simulink model "TeamA_PAsqualo_R19b"  (R2019b)
settings: Solver=VariableStepAuto  StartTime=0.0  StopTime=stop_time  FixedStep=0.05  RelTol=1e-3
InitFcn:
  | main_init
values from neighbouring files (symbols this model uses):
  a1 = rho * D^4 * alpha1    (= 0.000388302366464)    [data_current.m]    (also in main_init.m)
  a2 = -rho * D^3 * alpha2 * (1 - omega)    (= 0.0037030698432)    [data_current.m]    (also in main_init.m)
  ag = [Ax Ay Az]'    [init_modello.m]
  alpha1 = 0.0113    [data_current.m]    (also in main_init.m)
  alpha2 = -0.0091    [data_current.m]    (also in main_init.m)
  areaOfInterestCorner = [42.317744;10.915136; 0]    [init_controllo.m]    (also in missionA.m = [42.317744)
  bg = [Bx By Bz]'    [init_modello.m]
  cd_pitch = 0.7    [init_modello.m]
  cd_roll = 0.04    [init_modello.m]
  cd_x = 0.4    [init_modello.m]
  cd_y = 1    [init_modello.m]
  cd_yaw = 0.7    [init_modello.m]
  cd_z = 1    [init_modello.m]
  cg = [Cx Cy Cz]'    [init_modello.m]
  D = 0.076    [data_current.m]    (also in main_init.m)
  dead_zone_limit = 31.5    [data_current.m]    (also in main_init.m)
  dg = [Dx Dy Dz]'    [init_modello.m]
  eg = [Ex Ey Ez]'    [init_modello.m]
  fg = [Fx Fy Fz]'    [init_modello.m]
  g = 9.81    [init_modello.m]
  galleggiamento = 66.5386    [init_controllo.m]
  gg = [Gx Gy Gz]'    [init_modello.m]
  H0 = 0    [init_modello.m]
  init_position = [pointP(1),pointP(2),0.15,0,0,deg2rad(angle)]'    [appunti.m]    (also in init_modello.m = [pointP(1),pointP(2),0.15,0,0,deg2rad(alpha)]')
  init_velocity = [0 0 0 0 0 0]'    [init_modello.m]
  initial_state_cov = blkdiag(diag(cov_gps(1,1:2)), cov_depth*eye(n_state_filter-2))    [init_navigazione.m]
  Ixx = 0.93304097392    [init_modello.m]
  Ixy = 0    [init_modello.m]
  Ixz = 0    [init_modello.m]
  Iyy = 25.58745481378    (= 25.5874548138)    [init_modello.m]
  Iyz = 0    [init_modello.m]
  Izz = 25.58745481378    (= 25.5874548138)    [init_modello.m]
  K_i_heave_div = 20    [init_controllo.m]
  K_i_heave_pos = 1    [init_controllo.m]
  K_i_heave_surf = 20    [init_controllo.m]
  K_i_heave_trans = 5    [init_controllo.m]
  K_i_heave_turn = 5    [init_controllo.m]
  K_i_pitch_div = 0    [init_controllo.m]
  K_i_pitch_pos = 0.1*0    (= 0)    [init_controllo.m]
  K_i_pitch_surf = 0    [init_controllo.m]
  K_i_pitch_trans = 0    [init_controllo.m]
  K_i_pitch_turn = 0    [init_controllo.m]
  K_i_roll_div = 0    [init_controllo.m]
  K_i_roll_pos = 0.1*0    (= 0)    [init_controllo.m]
  K_i_roll_surf = 1    [init_controllo.m]
  K_i_roll_trans = 0    [init_controllo.m]
  K_i_roll_turn = 0    [init_controllo.m]
  K_i_surge_div = 3    [init_controllo.m]
  K_i_surge_pos = 0.1679*30    (= 5.037)    [init_controllo.m]
  K_i_surge_surf = 3    [init_controllo.m]
  K_i_surge_trans = 0.1679*15    (= 2.5185)    [init_controllo.m]
  K_i_surge_turn = 0.1679*60    (= 10.074)    [init_controllo.m]
  K_i_sway_div = 6    [init_controllo.m]
  K_i_sway_pos = 5    [init_controllo.m]
  K_i_sway_surf = 3    [init_controllo.m]
  K_i_sway_trans = 2    [init_controllo.m]
  K_i_sway_turn = 50    [init_controllo.m]
  K_i_yaw_div = 0    [init_controllo.m]
  K_i_yaw_pos = 1    [init_controllo.m]
  K_i_yaw_surf = 0    [init_controllo.m]
  K_i_yaw_trans = 20    [init_controllo.m]
  K_p_heave_div = 200    [init_controllo.m]
  K_p_heave_pos = 320    [init_controllo.m]
  K_p_heave_surf = 200    [init_controllo.m]
  K_p_heave_trans = 170    [init_controllo.m]
  K_p_heave_turn = 170    [init_controllo.m]
  K_p_phi_div = 0.15    [init_controllo.m]
  K_p_phi_pos = 1*0.1    (= 0.1)    [init_controllo.m]
  K_p_phi_surf = 0.15    [init_controllo.m]
  K_p_phi_trans = 0.1    [init_controllo.m]
  K_p_phi_turn = 0.1    [init_controllo.m]
  K_p_pitch_div = 50    [init_controllo.m]
  K_p_pitch_pos = 25    [init_controllo.m]
  K_p_pitch_surf = 50    [init_controllo.m]
  K_p_pitch_trans = 25    [init_controllo.m]
  K_p_pitch_turn = 25    [init_controllo.m]
  K_p_psi_div = 0.3    [init_controllo.m]
  K_p_psi_pos = 0.25    [init_controllo.m]
  K_p_psi_surf = 0.3    [init_controllo.m]
  K_p_psi_trans = 0.2    [init_controllo.m]
  K_p_roll_div = 10    [init_controllo.m]
  K_p_roll_pos = 0.1*40    (= 4)    [init_controllo.m]
  K_p_roll_surf = 10    [init_controllo.m]
  K_p_roll_trans = 0.1*40    (= 4)    [init_controllo.m]
  K_p_roll_turn = 4    [init_controllo.m]
  K_p_surge_div = 80    [init_controllo.m]
  K_p_surge_pos = 13.7782*2.5    (= 34.4455)    [init_controllo.m]
  K_p_surge_surf = 80    [init_controllo.m]
  K_p_surge_trans = 20    [init_controllo.m]
  K_p_surge_turn = 150    [init_controllo.m]
  K_p_sway_div = 100    [init_controllo.m]
  K_p_sway_pos = 90    [init_controllo.m]
  K_p_sway_surf = 80    [init_controllo.m]
  K_p_sway_trans = 80    [init_controllo.m]
  K_p_sway_turn = 200    [init_controllo.m]
  K_p_th_div = 0.3    [init_controllo.m]
  K_p_th_pos = 0.1    [init_controllo.m]
  K_p_th_surf = 0.3    [init_controllo.m]
  K_p_th_trans = 0.1    [init_controllo.m]
  K_p_th_turn = 0.1    [init_controllo.m]
  K_p_x_div = 0.12    [init_controllo.m]
  K_p_x_pos = 0.12    [init_controllo.m]
  K_p_x_surf = 0.12    [init_controllo.m]
  K_p_y_div = 0.6    [init_controllo.m]
  K_p_y_pos = 0.34    [init_controllo.m]
  K_p_y_surf = 0.1    [init_controllo.m]
  K_p_y_trans = 0.3    [init_controllo.m]
  K_p_y_turn = 0.3    [init_controllo.m]
  K_p_yaw_div = 70    [init_controllo.m]
  K_p_yaw_pos = 20    [init_controllo.m]
  K_p_yaw_surf = 70    [init_controllo.m]
  K_p_yaw_trans = 160    [init_controllo.m]
  K_p_z_div = 0.35    [init_controllo.m]
  K_p_z_pos = 0.2    [init_controllo.m]
  K_p_z_surf = 0.35    [init_controllo.m]
  K_p_z_trans = 0.10    (= 0.1)    [init_controllo.m]
  K_p_z_turn = 0.1    [init_controllo.m]
  Kadd = 0    [init_modello.m]
  m = 100    [init_modello.m]    (also in retta.m = p2-p1)
  Madd = -((((1/5)*(b^2-a^2)^2))*(alpha_0-beta_0))/((((2*(b^2-a^2)^2))+(b^2-a^2)^2)*(alpha_0-beta_0)*m)    [init_modello.m]
  ... (+59 more)
undefined symbols (not defined in the file or in its folder): DiscIntNeverNeededParam, initial_state
libraries: simulink x2, vrlib x1
(part 1 of 6)
settings Model: PauseTimes=1  PacingRate=5  Creator=User  LastModifiedBy=tolom

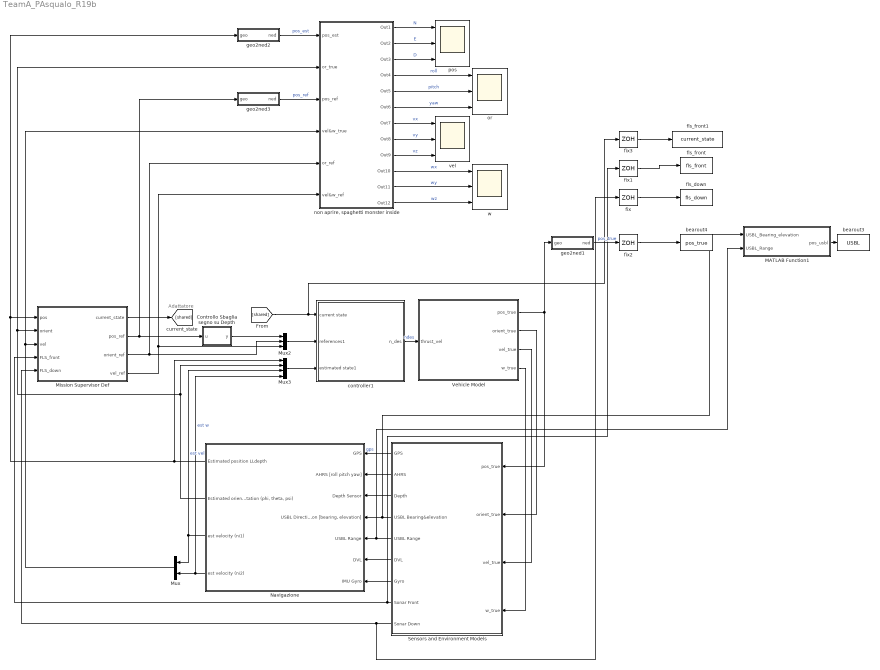
== system TeamA_PAsqualo_R19b ==
  note: Adattatore
  Controllo Sbaglia segno su Depth : MATLAB Function  TreatAsAtomicUnit=on
  MATLAB Function1 : MATLAB Function  TreatAsAtomicUnit=on
  Mission Supervisor Def : Subsystem
  Mux : Mux  Inputs=2
  Mux2 : Mux  Inputs=3
  Mux3 : Mux
  Navigazione : Subsystem
  "Sensors and Environment Models " : Subsystem
  Vehicle Model : Subsystem
  bearout3 : ToWorkspace  VariableName=USBL  SaveFormat=Structure With Time  SampleTime=-1
      settings: Save2DSignal=2-D array (concatenate along first dimension)
  bearout4 : ToWorkspace  VariableName=pos_true  SaveFormat=Structure With Time  SampleTime=-1
      settings: Save2DSignal=2-D array (concatenate along first dimension)
  controller1 : Subsystem
  fix{,1..3} (4 alike) : ZeroOrderHold  SampleTime=ts_filter
  fls_down : ToWorkspace  VariableName=fls_down  SaveFormat=Structure With Time  SampleTime=-1
      settings: Save2DSignal=2-D array (concatenate along first dimension)
  fls_front : ToWorkspace  VariableName=fls_front  SaveFormat=Structure With Time  SampleTime=-1
      settings: Save2DSignal=2-D array (concatenate along first dimension)
  fls_front1 : ToWorkspace  VariableName=current_state  SaveFormat=Structure With Time  SampleTime=-1
      settings: Save2DSignal=2-D array (concatenate along first dimension)
  geo2ned1 : MATLAB Function  TreatAsAtomicUnit=on
  geo2ned2 : MATLAB Function  TreatAsAtomicUnit=on
  geo2ned3 : MATLAB Function  TreatAsAtomicUnit=on
  "non aprire, spaghetti monster inside" : Subsystem
  or : Scope  NumInputPorts=3
  pos : Scope  NumInputPorts=3
  vel : Scope  NumInputPorts=3
  w : Scope  NumInputPorts=3
  wires:
  Mission Supervisor Def/4(vel_ref) -> "non aprire, spaghetti monster inside"/6(vel&w_ref), Mux2/3
  Mission Supervisor Def/3(orient_ref) -> "non aprire, spaghetti monster inside"/5(or_ref), Mux2/2
  Mission Supervisor Def/1(current_state) -> [shared]
  "Sensors and Environment Models "/8(Sonar Front) -> Mission Supervisor Def/4(FLS_front), fix1/1
  Vehicle Model/3(vel_true) -> "Sensors and Environment Models "/3(vel_true)
  Vehicle Model/4(w_true) -> "Sensors and Environment Models "/4(w_true)
  Mission Supervisor Def/2(pos_ref) -> geo2ned3/1(geo), Controllo Sbaglia segno su Depth/1(u)
  [shared] -> fix3/1, controller1/1(current state)
  Mux3/1 -> controller1/3(estimated state1)
  controller1/1(n_des) -> Vehicle Model/1(thrust_vel)  "ndes"
  "Sensors and Environment Models "/9(Sonar Down) -> Mission Supervisor Def/5(FLS_down), fix/1
  Vehicle Model/1(pos_true) -> "Sensors and Environment Models "/1(pos_true), geo2ned1/1(geo)
  Vehicle Model/2(orient_true) -> "Sensors and Environment Models "/2(orient_true)
  Navigazione/1(Estimated position LLdepth) -> Mux3/1, Mission Supervisor Def/1(pos), geo2ned2/1(geo)
  Navigazione/2("Estimated orientation (phi, theta, psi)") -> Mux3/2, Mission Supervisor Def/2(orient), "non aprire, spaghetti monster inside"/2(or_true)
  Navigazione/3(est velocity (ni1)) -> Mux/1, Mux3/3  "est vel"
  Navigazione/4(est velocity (ni2)) -> Mux3/4, Mux/2  "est w"
  Mux/1 -> Mission Supervisor Def/3(vel), "non aprire, spaghetti monster inside"/4(vel&w_true)
  geo2ned1/1(ned) -> fix2/1  "pos_true"
  MATLAB Function1/1(pos_usbl) -> bearout3/1
  "Sensors and Environment Models "/4(USBL Bearing&elevation) -> MATLAB Function1/1(USBL_Bearing_elevation), Navigazione/4("USBL Direction [bearing, elevation]")
  "Sensors and Environment Models "/5(USBL Range) -> MATLAB Function1/2(USBL_Range), Navigazione/5(USBL Range)
  "Sensors and Environment Models "/6(DVL) -> Navigazione/6(DVL)
  "Sensors and Environment Models "/7(Gyro) -> Navigazione/7(IMU Gyro)
  "Sensors and Environment Models "/3(Depth) -> Navigazione/3(Depth Sensor)
  "Sensors and Environment Models "/1(GPS) -> Navigazione/1(GPS)  "gps"
  "Sensors and Environment Models "/2(AHRS) -> Navigazione/2(AHRS [roll pitch yaw])
  "non aprire, spaghetti monster inside"/1(Out1) -> pos/1  "N"
  "non aprire, spaghetti monster inside"/2(Out2) -> pos/2  "E"
  "non aprire, spaghetti monster inside"/3(Out3) -> pos/3  "D"
  "non aprire, spaghetti monster inside"/4(Out4) -> or/1  "roll"
  "non aprire, spaghetti monster inside"/5(Out5) -> or/2  "pitch"
  "non aprire, spaghetti monster inside"/6(Out6) -> or/3  "yaw"
  "non aprire, spaghetti monster inside"/7(Out7) -> vel/1  "vx"
  "non aprire, spaghetti monster inside"/8(Out8) -> vel/2  "vy"
  "non aprire, spaghetti monster inside"/10(Out10) -> w/1  "wx"
  "non aprire, spaghetti monster inside"/11(Out11) -> w/2  "wy"
  "non aprire, spaghetti monster inside"/12(Out12) -> w/3  "wz"
  "non aprire, spaghetti monster inside"/9(Out9) -> vel/3  "vz"
  geo2ned2/1(ned) -> "non aprire, spaghetti monster inside"/1(pos_est)  "pos_est"
  geo2ned3/1(ned) -> "non aprire, spaghetti monster inside"/3(pos_ref)  "pos_ref"
  Mux2/1 -> controller1/2(references1)
  Controllo Sbaglia segno su Depth/1(y) -> Mux2/1
  fix/1 -> fls_down/1
  fix1/1 -> fls_front/1
  fix2/1 -> bearout4/1
  fix3/1 -> fls_front1/1

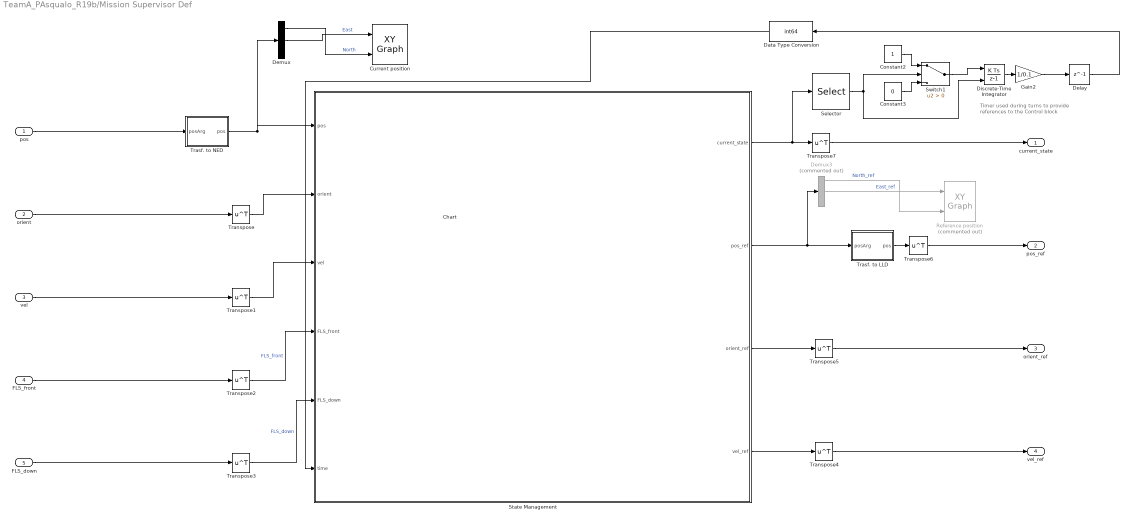
== system TeamA_PAsqualo_R19b/Mission Supervisor Def ==
  note: Timer used during turns to
      | provide references to the Control block
  pos : Inport
  orient : Inport  Port=2  PortDimensions=[3 1]
  vel : Inport  Port=3  PortDimensions=[6 1]
  FLS_front : Inport  Port=4  PortDimensions=1
  FLS_down : Inport  Port=5  PortDimensions=1
  Chart : Stateflow chart  TreatAsAtomicUnit=on
  Constant2 : Constant
  Constant3 : Constant  Value=0
  Current position : simulink/Sinks/XY Graph  xmin=0  xmax=150  ymin=0  ymax=150  st=-1
  Data Type Conversion : DataTypeConversion  OutDataTypeStr=int64
  Delay : Delay  DelayLength=1  SampleTime=0.1
  Demux : Demux  Outputs=3
  Demux3 : Demux  Commented=on  Outputs=3
  Discrete-Time Integrator : DiscreteIntegrator  ExternalReset=falling  SampleTime=0.1  ICPrevOutput=DiscIntNeverNeededParam  ICPrevScaledInput=DiscIntNeverNeededParam
  Gain2 : Gain  Gain=1/0.1
  Reference position : simulink/Sinks/XY Graph  Commented=on  xmin=0  xmax=150  ymin=0  ymax=150  st=-1
  Selector : Selector  InputPortWidth=8  IndexOptions=Index vector (dialog)  Indices=4  OutputSizes=1
  State Management : Stateflow chart  TreatAsAtomicUnit=on
  Switch1 : Switch  Criteria=u2 > Threshold
  Transpose{,1..7} (8 alike) : Math  Operator=transpose  SaturateOnIntegerOverflow=on
  Trasf. to LLD : MATLAB Function  TreatAsAtomicUnit=on
  Trasf. to NED : MATLAB Function  TreatAsAtomicUnit=on
  current_state : Outport
  pos_ref : Outport  Port=2
  orient_ref : Outport  Port=3
  vel_ref : Outport  Port=4  PortDimensions=[6 1]
  wires:
  Transpose3/1 -> State Management/5(FLS_down)  "FLS_down"
  FLS_front/1 -> Transpose2/1
  Transpose5/1 -> orient_ref/1
  orient/1 -> Transpose/1
  vel/1 -> Transpose1/1
  Transpose4/1 -> vel_ref/1
  FLS_down/1 -> Transpose3/1
  Demux/1 -> Current position/2  "North"
  Demux/2 -> Current position/1  "East"
  Transpose/1 -> State Management/2(orient)
  Transpose1/1 -> State Management/3(vel)
  Transpose2/1 -> State Management/4(FLS_front)  "FLS_front"
  Demux3/1 -> Reference position/2  "North_ref"
  Demux3/2 -> Reference position/1  "East_ref"
  State Management/3(orient_ref) -> Transpose5/1
  State Management/4(vel_ref) -> Transpose4/1
  pos/1 -> Trasf. to NED/1(posArg)
  State Management/2(pos_ref) -> Trasf. to LLD/1(posArg), Demux3/1
  Trasf. to LLD/1(pos) -> Transpose6/1
  Trasf. to NED/1(pos) -> Demux/1, State Management/1(pos)
  Transpose6/1 -> pos_ref/1
  Transpose7/1 -> current_state/1
  Discrete-Time Integrator/1 -> Gain2/1
  Selector/1 -> Discrete-Time Integrator/2, Switch1/2
  Switch1/1 -> Discrete-Time Integrator/1
  Constant3/1 -> Switch1/3
  Constant2/1 -> Switch1/1
  Data Type Conversion/1 -> State Management/6(time)
  Gain2/1 -> Delay/1
  Delay/1 -> Data Type Conversion/1
  State Management/1(current_state) -> Selector/1, Transpose7/1

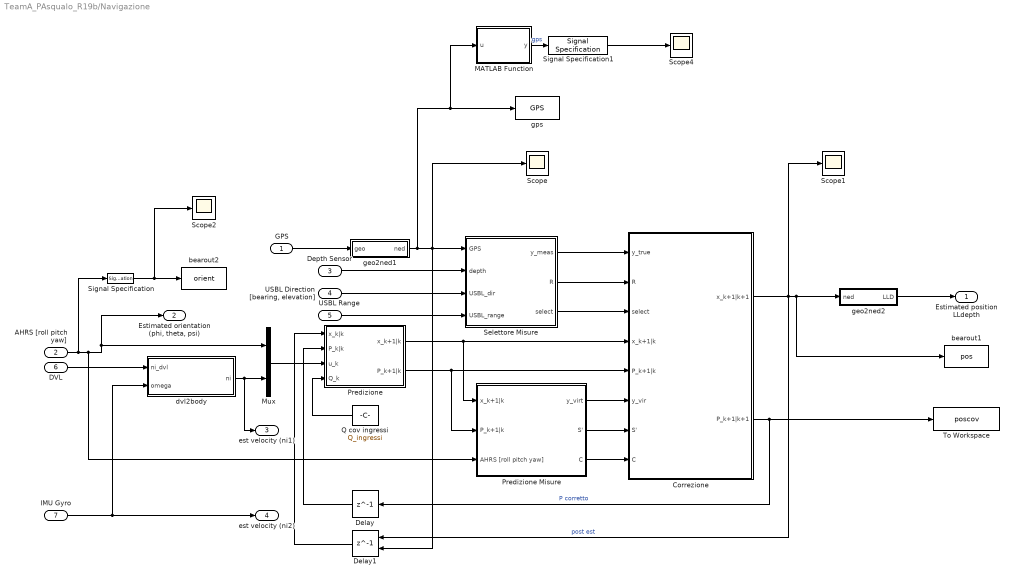
== system TeamA_PAsqualo_R19b/Navigazione ==
  GPS : Inport  PortDimensions=[3 1]
  AHRS [roll pitch yaw] : Inport  Port=2  PortDimensions=[3 1]
  Depth Sensor : Inport  Port=3  PortDimensions=[1 1]
  "USBL Direction [bearing, elevation]" : Inport  Port=4  PortDimensions=[2 1]
  USBL Range : Inport  Port=5  PortDimensions=[1 1]
  DVL : Inport  Port=6  PortDimensions=[3 1]
  IMU Gyro : Inport  Port=7  PortDimensions=[3 1]
  Correzione : Subsystem
  Delay : Delay  DelayLength=1  InitialCondition=initial_state_cov  SampleTime=ts_filter
  Delay1 : Delay  DelayLength=1  InitialConditionSource=Input port  InitialCondition=initial_state  SampleTime=ts_filter
      settings: InputPortMap=u0,p4
  MATLAB Function : MATLAB Function  TreatAsAtomicUnit=on
  Mux : Mux  Inputs=2
  Predizione : Subsystem
  Predizione Misure : Subsystem
  Q cov ingressi : Constant  Value=Q_ingressi
  Scope{,1..2,4} (4 alike) : Scope
  Selettore Misure : Subsystem
  Signal Specification : SignalSpecification  Dimensions=[3,1]
  Signal Specification1 : SignalSpecification  Dimensions=1
  To Workspace : ToWorkspace  VariableName=poscov  SaveFormat=Structure With Time  SampleTime=-1
  bearout1 : ToWorkspace  VariableName=pos  SaveFormat=Structure With Time  SampleTime=-1
      settings: Save2DSignal=2-D array (concatenate along first dimension)
  bearout2 : ToWorkspace  VariableName=orient  SaveFormat=Structure With Time  SampleTime=-1
      settings: Save2DSignal=2-D array (concatenate along first dimension)
  dvl2body : MATLAB Function  TreatAsAtomicUnit=on
  geo2ned1 : MATLAB Function  TreatAsAtomicUnit=on
  geo2ned2 : MATLAB Function  TreatAsAtomicUnit=on
  gps : ToWorkspace  VariableName=GPS  SaveFormat=Structure With Time  SampleTime=-1
      settings: Save2DSignal=2-D array (concatenate along first dimension)
  Estimated position LLdepth : Outport
  "Estimated orientation (phi, theta, psi)" : Outport  Port=2
  est velocity (ni1) : Outport  Port=3
  est velocity (ni2) : Outport  Port=4
  wires:
  Delay1/1 -> Predizione/1(x_k|k)
  Selettore Misure/2(R) -> Correzione/2(R)
  Selettore Misure/1(y_meas) -> Correzione/1(y_true)
  USBL Range/1 -> Selettore Misure/4(USBL_range)
  DVL/1 -> dvl2body/1(ni_dvl)
  Correzione/2(P_k+1|k+1) -> Delay/1, To Workspace/1  "P corretto"
  Predizione Misure/3(C) -> Correzione/8(C)
  Mux/1 -> Predizione/3(u_k)
  GPS/1 -> geo2ned1/1(geo)
  dvl2body/1(ni) -> est velocity (ni1)/1, Mux/2
  Delay/1 -> Predizione/2(P_k|k)
  Selettore Misure/3(select) -> Correzione/3(select)
  Depth Sensor/1 -> Selettore Misure/2(depth)
  Predizione Misure/2(S') -> Correzione/7(S')
  "USBL Direction [bearing, elevation]"/1 -> Selettore Misure/3(USBL_dir)
  Q cov ingressi/1 -> Predizione/4(Q_k)
  Predizione/1(x_k+1|k) -> Predizione Misure/1(x_k+1|k), Correzione/4(x_k+1|k)
  Predizione Misure/1(y_virt) -> Correzione/6(y_vir)
  AHRS [roll pitch yaw]/1 -> Predizione Misure/3(AHRS [roll pitch yaw]), Mux/1, "Estimated orientation (phi, theta, psi)"/1, Signal Specification/1
  Predizione/2(P_k+1|k) -> Predizione Misure/2(P_k+1|k), Correzione/5(P_k+1|k)
  IMU Gyro/1 -> est velocity (ni2)/1, dvl2body/2(omega)
  geo2ned2/1(LLD) -> Estimated position LLdepth/1
  Correzione/1(x_k+1|k+1) -> Scope1/1, bearout1/1, geo2ned2/1(ned), Delay1/1  "post est"
  Signal Specification/1 -> Scope2/1, bearout2/1
  geo2ned1/1(ned) -> MATLAB Function/1(u), gps/1, Scope/1, Delay1/2, Selettore Misure/1(GPS)
  MATLAB Function/1(y) -> Signal Specification1/1  "gps"
  Signal Specification1/1 -> Scope4/1

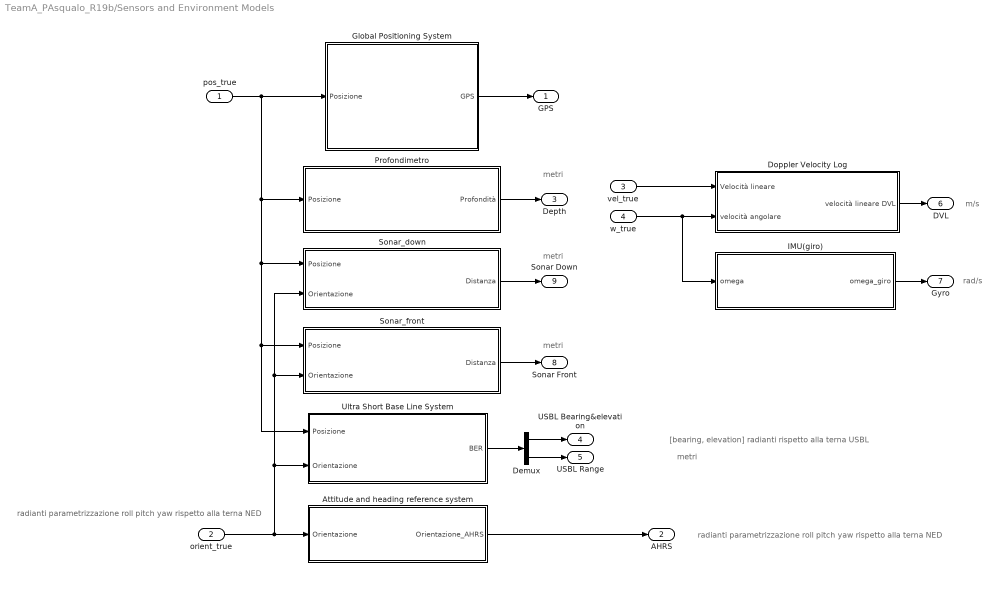
== system TeamA_PAsqualo_R19b/Sensors and Environment Models  ==
  note: radianti parametrizzazione roll pitch yaw rispetto alla terna NED
  note: m/s
  note: metri
  note: [bearing, elevation] radianti rispetto alla terna USBL
  note: rad/s
  note: metri
  note: metri
  note: metri
  note: radianti parametrizzazione roll pitch yaw rispetto alla terna NED
  pos_true : Inport
  orient_true : Inport  Port=2
  vel_true : Inport  Port=3
  w_true : Inport  Port=4
  Attitude and heading reference system : Subsystem
  Demux : Demux  Outputs=2
  Doppler Velocity Log : Subsystem
  Global Positioning System : Subsystem
  IMU(giro) : Subsystem
  Profondimetro : Subsystem
  Sonar_down : Subsystem
  Sonar_front : Subsystem
  Ultra Short Base Line System : Subsystem
  GPS : Outport
  AHRS : Outport  Port=2
  Depth : Outport  Port=3
  USBL Bearing&elevation : Outport  Port=4
  USBL Range : Outport  Port=5
  DVL : Outport  Port=6
  Gyro : Outport  Port=7
  Sonar Front : Outport  Port=8
  Sonar Down : Outport  Port=9
  wires:
  IMU(giro)/1(omega_giro) -> Gyro/1
  vel_true/1 -> Doppler Velocity Log/1(Velocità lineare)
  pos_true/1 -> Ultra Short Base Line System/1(Posizione), Sonar_front/1(Posizione), Sonar_down/1(Posizione), Profondimetro/1(Posizione), Global Positioning System/1(Posizione)
  orient_true/1 -> Attitude and heading reference system/1(Orientazione), Ultra Short Base Line System/2(Orientazione), Sonar_down/2(Orientazione), Sonar_front/2(Orientazione)
  w_true/1 -> IMU(giro)/1(omega), Doppler Velocity Log/2(velocità angolare)
  Sonar_down/1(Distanza) -> Sonar Down/1
  Profondimetro/1(Profondità) -> Depth/1
  Demux/2 -> USBL Range/1
  Doppler Velocity Log/1(velocità lineare DVL) -> DVL/1
  Sonar_front/1(Distanza) -> Sonar Front/1
  Global Positioning System/1(GPS) -> GPS/1
  Demux/1 -> USBL Bearing&elevation/1
  Attitude and heading reference system/1(Orientazione_AHRS) -> AHRS/1
  Ultra Short Base Line System/1(BER) -> Demux/1

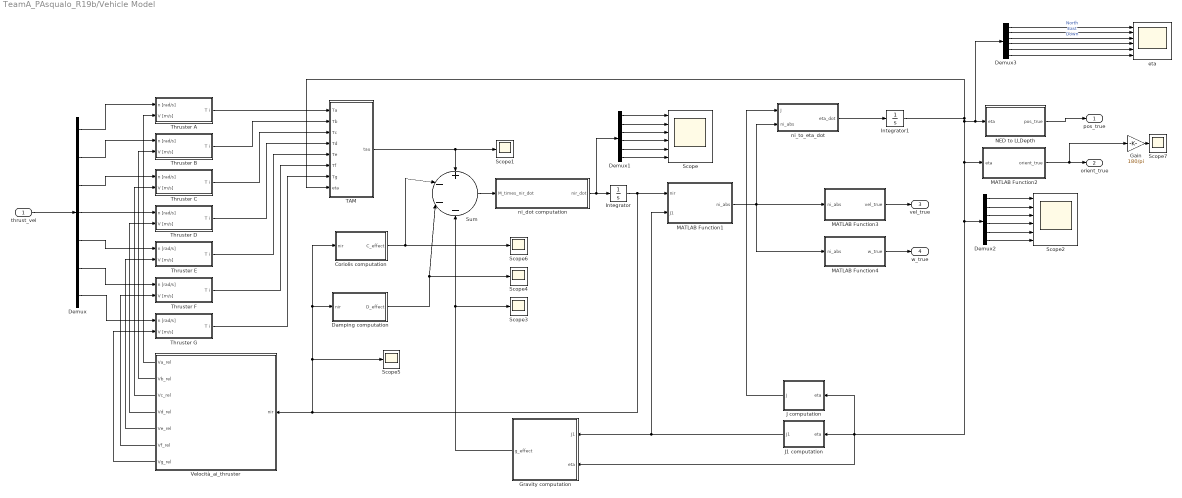
== system TeamA_PAsqualo_R19b/Vehicle Model ==
  thrust_vel : Inport
  Coriolis computation : MATLAB Function  TreatAsAtomicUnit=on
  Damping computation : MATLAB Function  TreatAsAtomicUnit=on
  Demux : Demux  Outputs=7
  Demux1 : Demux  Outputs=6
  Demux2 : Demux  Outputs=6
  Demux3 : Demux  Outputs=6
  Gain : Gain  Gain=180/pi
  Gravity computation : MATLAB Function  TreatAsAtomicUnit=on
  Integrator : Integrator  InitialCondition=init_velocity  ContinuousStateAttributes='velocity'
  Integrator1 : Integrator  InitialCondition=init_position  ContinuousStateAttributes='position'
  J computation : MATLAB Function  TreatAsAtomicUnit=on
  J1 computation : MATLAB Function  TreatAsAtomicUnit=on
  MATLAB Function1 : MATLAB Function  TreatAsAtomicUnit=on
  MATLAB Function2 : MATLAB Function  TreatAsAtomicUnit=on
  MATLAB Function3 : MATLAB Function  TreatAsAtomicUnit=on
  MATLAB Function4 : MATLAB Function  TreatAsAtomicUnit=on
  NED to LLDepth : MATLAB Function  TreatAsAtomicUnit=on
  Scope : Scope  NumInputPorts=6
  Scope{1,3..7} (6 alike) : Scope
  Scope2 : Scope  NumInputPorts=6
  Sum : Sum  Inputs=+---
  TAM : MATLAB Function
  Thruster A : Subsystem
  Thruster B : Subsystem
  Thruster C : Subsystem
  Thruster D : Subsystem
  Thruster E : Subsystem
  Thruster F : Subsystem
  Thruster G : Subsystem
  Velocità_ai_thruster : MATLAB Function  TreatAsAtomicUnit=on
  eta : Scope  NumInputPorts=6
  ni_dot computation : MATLAB Function  TreatAsAtomicUnit=on
  ni_to_eta_dot : MATLAB Function  TreatAsAtomicUnit=on
  pos_true : Outport
  orient_true : Outport  Port=2
  vel_true : Outport  Port=3
  w_true : Outport  Port=4
  wires:
  Demux/3 -> Thruster C/1(n [rad/s])
  Thruster A/1(T i) -> TAM/1(Ta)
  Thruster G/1(T i) -> TAM/7(Tg)
  Sum/1 -> ni_dot computation/1(M_times_nir_dot)
  Velocità_ai_thruster/7(Vg_rel) -> Thruster G/2(V [m/s])
  Velocità_ai_thruster/3(Vc_rel) -> Thruster C/2(V [m/s])
  Thruster C/1(T i) -> TAM/3(Tc)
  MATLAB Function3/1(vel_true) -> vel_true/1
  Gravity computation/1(g_effect) -> Sum/4, Scope3/1
  Demux/6 -> Thruster F/1(n [rad/s])
  MATLAB Function4/1(w_true) -> w_true/1
  J1 computation/1(J1) -> Gravity computation/1(J1), MATLAB Function1/2(J1)
  Thruster F/1(T i) -> TAM/6(Tf)
  Integrator/1 -> Scope5/1, Coriolis computation/1(nir), Damping computation/1(nir), Velocità_ai_thruster/1(nir), MATLAB Function1/1(nir)
  Velocità_ai_thruster/4(Vd_rel) -> Thruster D/2(V [m/s])
  Velocità_ai_thruster/6(Vf_rel) -> Thruster F/2(V [m/s])
  ni_dot computation/1(nir_dot) -> Demux1/1, Integrator/1
  Velocità_ai_thruster/2(Vb_rel) -> Thruster B/2(V [m/s])
  MATLAB Function1/1(ni_abs) -> ni_to_eta_dot/2(ni_abs), MATLAB Function3/1(ni_abs), MATLAB Function4/1(ni_abs)
  Velocità_ai_thruster/1(Va_rel) -> Thruster A/2(V [m/s])
  Demux/4 -> Thruster D/1(n [rad/s])
  Thruster E/1(T i) -> TAM/5(Te)
  Thruster B/1(T i) -> TAM/2(Tb)
  Demux/2 -> Thruster B/1(n [rad/s])
  TAM/1(tau) -> Sum/1, Scope1/1
  ni_to_eta_dot/1(eta_dot) -> Integrator1/1
  MATLAB Function2/1(orient_true) -> Gain/1, orient_true/1
  Demux/1 -> Thruster A/1(n [rad/s])
  Velocità_ai_thruster/5(Ve_rel) -> Thruster E/2(V [m/s])
  Demux/5 -> Thruster E/1(n [rad/s])
  NED to LLDepth/1(pos_true) -> pos_true/1
  Thruster D/1(T i) -> TAM/4(Td)
  J computation/1(J) -> ni_to_eta_dot/1(J)
  thrust_vel/1 -> Demux/1
  Demux/7 -> Thruster G/1(n [rad/s])
  Damping computation/1(D_effect) -> Sum/3, Scope4/1
  Coriolis computation/1(C_effect) -> Sum/2, Scope6/1
  Demux1/1 -> Scope/1
  Demux1/2 -> Scope/2
  Demux1/3 -> Scope/3
  Demux1/5 -> Scope/5
  Demux1/6 -> Scope/6
  Demux1/4 -> Scope/4
  Demux2/6 -> Scope2/6
  Demux2/5 -> Scope2/5
  Demux2/3 -> Scope2/3
  Demux2/2 -> Scope2/2
  Demux2/4 -> Scope2/4
  Demux2/1 -> Scope2/1
  Demux3/3 -> eta/3  "Down"
  Demux3/1 -> eta/1  "North"
  Demux3/2 -> eta/2  "East"
  Integrator1/1 -> TAM/8(eta), Demux3/1, NED to LLDepth/1(eta), J computation/1(eta), Gravity computation/2(eta), J1 computation/1(eta), Demux2/1, MATLAB Function2/1(eta)
  Demux3/4 -> eta/4
  Demux3/5 -> eta/5
  Demux3/6 -> eta/6
  Gain/1 -> Scope7/1

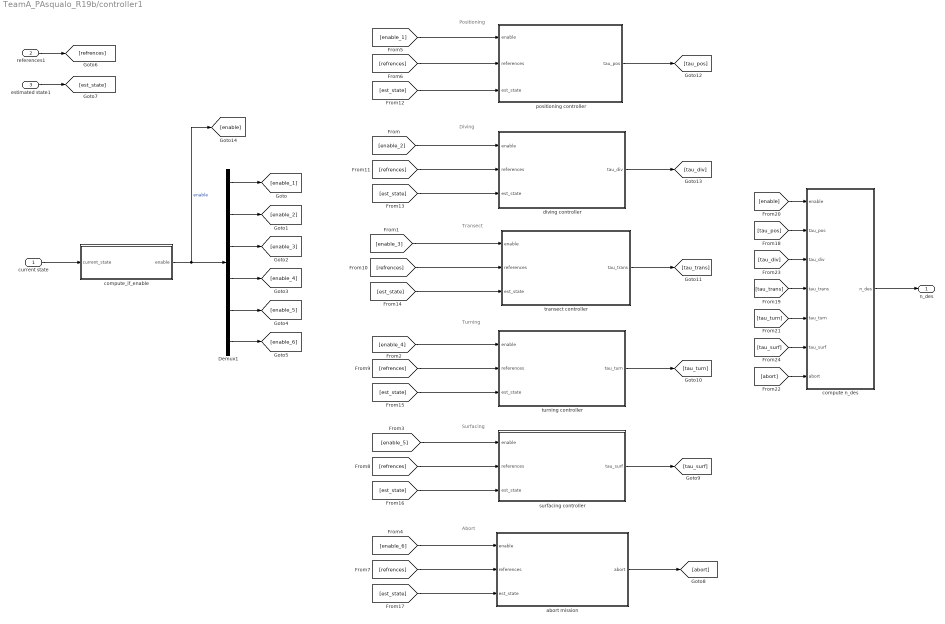
== system TeamA_PAsqualo_R19b/controller1 ==
  note: Diving
  note: Positioning
  note: Transect
  note: Abort
  note: Surfacing
  note: Turning
  current state : Inport
  references1 : Inport  Port=2
  estimated state1 : Inport  Port=3
  Demux1 : Demux  Outputs=6
  abort mission : Subsystem
  compute n_des : MATLAB Function  TreatAsAtomicUnit=on
  compute_if_enable : MATLAB Function  TreatAsAtomicUnit=on
  diving controller : Subsystem
  positioning controller : Subsystem
  surfacing controller : Subsystem
  transect controller : Subsystem
  turning controller : Subsystem
  n_des : Outport
  wires:
  [enable] -> compute n_des/1(enable)
  [enable_5] -> surfacing controller/1(enable)
  abort mission/1(abort) -> [abort]
  compute_if_enable/1(enable) -> [enable], Demux1/1  "enable"
  Demux1/3 -> [enable_3]
  Demux1/4 -> [enable_4]
  [tau_pos] -> compute n_des/2(tau_pos)
  [tau_surf] -> compute n_des/6(tau_surf)
  Demux1/5 -> [enable_5]
  Demux1/6 -> [enable_6]
  [refrences] -> diving controller/2(references)
  references1/1 -> [refrences]
  turning controller/1(tau_turn) -> [tau_turn]
  [enable_2] -> diving controller/1(enable)
  [enable_4] -> turning controller/1(enable)
  [est_state] -> abort mission/3(est_state)
  current state/1 -> compute_if_enable/1(current_state)
  [tau_turn] -> compute n_des/5(tau_turn)
  [enable_1] -> positioning controller/1(enable)
  [refrences] -> abort mission/2(references)
  Demux1/2 -> [enable_2]
  [est_state] -> turning controller/3(est_state)
  Demux1/1 -> [enable_1]
  [refrences] -> transect controller/2(references)
  diving controller/1(tau_div) -> [tau_div]
  [tau_trans] -> compute n_des/4(tau_trans)
  positioning controller/1(tau_pos) -> [tau_pos]
  [tau_div] -> compute n_des/3(tau_div)
  surfacing controller/1(tau_surf) -> [tau_surf]
  [abort] -> compute n_des/7(abort)
  [refrences] -> surfacing controller/2(references)
  [enable_3] -> transect controller/1(enable)
  [refrences] -> positioning controller/2(references)
  [refrences] -> turning controller/2(references)
  [enable_6] -> abort mission/1(enable)
  estimated state1/1 -> [est_state]
  [est_state] -> positioning controller/3(est_state)
  [est_state] -> diving controller/3(est_state)
  transect controller/1(tau_trans) -> [tau_trans]
  [est_state] -> transect controller/3(est_state)
  [est_state] -> surfacing controller/3(est_state)
  compute n_des/1(n_des) -> n_des/1

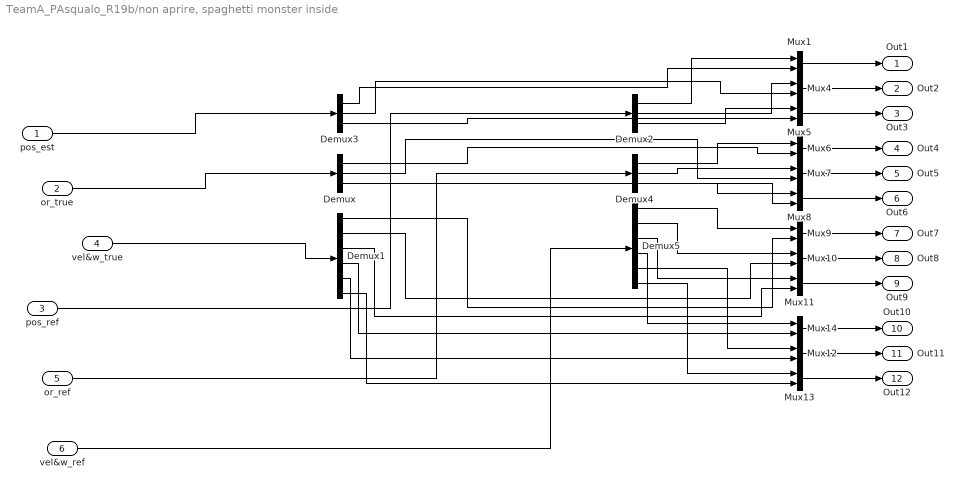
== system TeamA_PAsqualo_R19b/non aprire, spaghetti monster inside ==
  pos_est : Inport
  or_true : Inport  Port=2
  pos_ref : Inport  Port=3
  vel&w_true : Inport  Port=4
  or_ref : Inport  Port=5
  vel&w_ref : Inport  Port=6
  Demux{,2..4} (4 alike) : Demux  Outputs=3
  Demux1 : Demux  Outputs=6
  Demux5 : Demux  Outputs=6
  Mux{1,4..14} (12 alike) : Mux  Inputs=2
  Out1 : Outport
  Out2 : Outport  Port=2
  Out3 : Outport  Port=3
  Out4 : Outport  Port=4
  Out5 : Outport  Port=5
  Out6 : Outport  Port=6
  Out7 : Outport  Port=7
  Out8 : Outport  Port=8
  Out9 : Outport  Port=9
  Out10 : Outport  Port=10
  Out11 : Outport  Port=11
  Out12 : Outport  Port=12
  wires:
  Mux6/1 -> Out4/1
  Demux1/2 -> Mux10/2
  Demux1/4 -> Mux14/2
  Demux/2 -> Mux7/2
  Demux3/3 -> Mux5/2
  Mux8/1 -> Out6/1
  Demux5/5 -> Mux12/1
  Demux/1 -> Mux6/2
  Demux/3 -> Mux8/2
  Demux1/6 -> Mux13/2
  Demux5/4 -> Mux14/1
  Demux5/1 -> Mux9/1
  Demux1/3 -> Mux11/2
  Demux4/1 -> Mux6/1
  Demux4/3 -> Mux8/1
  Demux2/2 -> Mux4/1
  Demux5/2 -> Mux10/1
  Mux1/1 -> Out1/1
  Demux2/3 -> Mux5/1
  Demux1/1 -> Mux9/2
  Demux5/3 -> Mux11/1
  or_ref/1 -> Demux4/1
  Mux11/1 -> Out9/1
  Demux5/6 -> Mux13/1
  Demux3/2 -> Mux4/2
  Demux3/1 -> Mux1/2
  Demux2/1 -> Mux1/1
  Demux4/2 -> Mux7/1
  pos_ref/1 -> Demux2/1
  pos_est/1 -> Demux3/1
  Demux1/5 -> Mux12/2
  Mux4/1 -> Out2/1
  vel&w_true/1 -> Demux1/1
  Mux5/1 -> Out3/1
  Mux10/1 -> Out8/1
  Mux7/1 -> Out5/1
  Mux9/1 -> Out7/1
  or_true/1 -> Demux/1
  vel&w_ref/1 -> Demux5/1
  Mux12/1 -> Out11/1
  Mux13/1 -> Out12/1
  Mux14/1 -> Out10/1

== system TeamA_PAsqualo_R19b/Mission Supervisor Def/State Management/Movements.End ==
  note: Function used to stop the mission once
      | the vehicle is back at the starting point
  f : TriggerPort  TriggerType=function-call  VariantControl=(inherit)
      settings: CopyFcn=Stateflow.SLINSF.SimulinkMan.removeBlockPreDeleteFcn  PreDeleteFcn=Stateflow.SLINSF.SimulinkMan.unsafePredeleteFcn
  Constant : Constant
  Stop Simulation : Stop
  wires:
  Constant/1 -> Stop Simulation/1

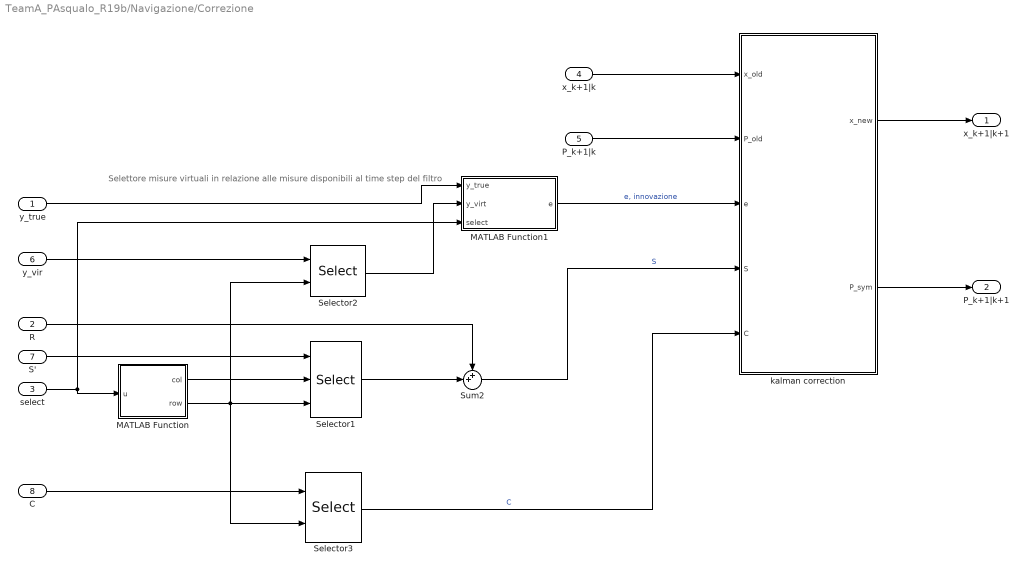
== system TeamA_PAsqualo_R19b/Navigazione/Correzione ==
  note: Selettore misure virtuali in relazione alle misure disponibili al time step del filtro
  y_true : Inport
  R : Inport  Port=2
  select : Inport  Port=3
  x_k+1|k : Inport  Port=4
  P_k+1|k : Inport  Port=5
  y_vir : Inport  Port=6
  S' : Inport  Port=7
  C : Inport  Port=8
  MATLAB Function : MATLAB Function  TreatAsAtomicUnit=on  SystemSampleTime=ts_filter
  MATLAB Function1 : MATLAB Function  TreatAsAtomicUnit=on
  Selector1 : Selector  NumberOfDimensions=2  InputPortWidth=3  IndexOptions=Index vector (port),Index vector (port)  Indices=[1 3],1  OutputSizes=1,1
  Selector2 : Selector  InputPortWidth=5  IndexOptions=Index vector (port)  Indices=[1 3]  OutputSizes=1
  Selector3 : Selector  NumberOfDimensions=2  InputPortWidth=3  IndexOptions=Select all,Index vector (port)  Indices=[1 3],1  OutputSizes=1,1
  Sum2 : Sum  Inputs=++|
  kalman correction : MATLAB Function  TreatAsAtomicUnit=on  SystemSampleTime=ts_filter
  x_k+1|k+1 : Outport
  P_k+1|k+1 : Outport  Port=2
  wires:
  Sum2/1 -> kalman correction/4(S)  "S"
  x_k+1|k/1 -> kalman correction/1(x_old)
  P_k+1|k/1 -> kalman correction/2(P_old)
  kalman correction/1(x_new) -> x_k+1|k+1/1
  kalman correction/2(P_sym) -> P_k+1|k+1/1
  y_true/1 -> MATLAB Function1/1(y_true)
  MATLAB Function1/1(e) -> kalman correction/3(e)  "e, innovazione"
  MATLAB Function/2(row) -> Selector3/2, Selector1/3, Selector2/2
  S'/1 -> Selector1/1
  Selector1/1 -> Sum2/2
  MATLAB Function/1(col) -> Selector1/2
  Selector2/1 -> MATLAB Function1/2(y_virt)
  y_vir/1 -> Selector2/1
  select/1 -> MATLAB Function/1(u), MATLAB Function1/3(select)
  C/1 -> Selector3/1
  Selector3/1 -> kalman correction/5(C)  "C"
  R/1 -> Sum2/1

== system TeamA_PAsqualo_R19b/Navigazione/Predizione ==
  x_k|k : Inport
  P_k|k : Inport  Port=2
  u_k : Inport  Port=3
  Q_k : Inport  Port=4
  predizione_propagate : MATLAB Function  TreatAsAtomicUnit=on  SystemSampleTime=ts_filter
  smart_mux : MATLAB Function  TreatAsAtomicUnit=on  SystemSampleTime=ts_filter
  x_k+1|k : Outport
  P_k+1|k : Outport  Port=2
  wires:
  Q_k/1 -> smart_mux/4(u_cov)
  x_k|k/1 -> smart_mux/1(x_mean)
  predizione_propagate/1(mean_new) -> x_k+1|k/1
  predizione_propagate/2(cov_new) -> P_k+1|k/1
  smart_mux/2(cov) -> predizione_propagate/2(cov)  "cov aumentata"
  smart_mux/1(mean) -> predizione_propagate/1(mean)  "stato aumentato"
  P_k|k/1 -> smart_mux/2(x_cov)
  u_k/1 -> smart_mux/3(u_mean)

== system TeamA_PAsqualo_R19b/Navigazione/Predizione Misure ==
  x_k+1|k : Inport
  P_k+1|k : Inport  Port=2
  AHRS [roll pitch yaw] : Inport  Port=3
  propagazione misura NED1 : MATLAB Function  TreatAsAtomicUnit=on  SystemSampleTime=ts_filter
  y_virt : Outport
  S' : Outport  Port=2
  C : Outport  Port=3
  wires:
  propagazione misura NED1/3(C) -> C/1
  propagazione misura NED1/1(y_virt) -> y_virt/1
  x_k+1|k/1 -> propagazione misura NED1/1(x)
  P_k+1|k/1 -> propagazione misura NED1/2(P)
  propagazione misura NED1/2(S_virt) -> S'/1
  AHRS [roll pitch yaw]/1 -> propagazione misura NED1/3(or)

== system TeamA_PAsqualo_R19b/Navigazione/Selettore Misure ==
  note: ymeas = 	lat
      | 			lon
      | 			bear
      | 			range
      | 			depth
  GPS : Inport
  depth : Inport  Port=2
  USBL_dir : Inport  Port=3
  USBL_range : Inport  Port=4
  Selettore misure : Subsystem
  Signal Specification : SignalSpecification  Dimensions=2
  Terminator : Terminator
  Terminator1 : Terminator
  dir_demux : Demux  Outputs=2
  gps_demux : Demux  Outputs=2
  y_meas : Outport
  R : Outport  Port=2
  select : Outport  Port=3
  wires:
  GPS/1 -> gps_demux/1
  Selettore misure/2(R) -> R/1
  Signal Specification/1 -> Selettore misure/1(GPS)
  gps_demux/2 -> Terminator1/1
  dir_demux/1 -> Selettore misure/3(USBL_bear)
  dir_demux/2 -> Terminator/1  "elev_term"
  gps_demux/1 -> Signal Specification/1
  USBL_range/1 -> Selettore misure/4(USBL_range)
  depth/1 -> Selettore misure/2(depth)
  USBL_dir/1 -> dir_demux/1
  Selettore misure/1(y_meas) -> y_meas/1
  Selettore misure/3(select) -> select/1

== system TeamA_PAsqualo_R19b/Sensors and Environment Models /Attitude and heading reference system ==
  note: rad
  Orientazione : Inport  SampleTime=Ts_ahrs
  Quantizer : Quantizer  QuantizationInterval=res_ahrs
  Random Number : RandomNumber  Variance=var_ahrs  Seed=[26; 78; 90]  SampleTime=Ts_ahrs  VectorParams1D=off
  Sum : Sum  Inputs=|++
  Orientazione_AHRS : Outport  VectorParamsAs1DForOutWhenUnconnected=off
  wires:
  Random Number/1 -> Sum/2
  Sum/1 -> Quantizer/1
  Orientazione/1 -> Sum/1
  Quantizer/1 -> Orientazione_AHRS/1

== system TeamA_PAsqualo_R19b/Sensors and Environment Models /Doppler Velocity Log ==
  note: distanza in terna body del sensore DVL dal centro di massa
  note: cross product
  note: m/s
  Velocità lineare : Inport  SampleTime=Ts_dvl
  velocità angolare : Inport  Port=2  SampleTime=Ts_dvl
  Constant : Constant  Value=p_dvl  VectorParams1D=off
  Cross Product : vrlib/Utilities/Cross Product
      settings: SourceProductBaseCode=VR
  Quantizer : Quantizer  QuantizationInterval=res_dvl
  Random Number : RandomNumber  Variance=var_dvl  Seed=[21, 68, 10]  SampleTime=Ts_dvl
  Sum : Sum  Inputs=|++
  Sum1 : Sum  Inputs=|++
  velocità lineare DVL : Outport  VectorParamsAs1DForOutWhenUnconnected=off
  wires:
  Sum/1 -> Quantizer/1
  Random Number/1 -> Sum/2
  velocità angolare/1 -> Cross Product/1
  Constant/1 -> Cross Product/2
  Velocità lineare/1 -> Sum1/1
  Cross Product/1 -> Sum1/2
  Sum1/1 -> Sum/1
  Quantizer/1 -> velocità lineare DVL/1

== system TeamA_PAsqualo_R19b/Sensors and Environment Models /Global Positioning System ==
  note: profondità [metri]
  note: GPS funzionante
  note: metri
  note: GPS non funzionante
  Posizione : Inport  SampleTime=Ts_gps
  Constant : Constant  Value=[0;0;0]  VectorParams1D=off
  MATLAB Function : MATLAB Function  TreatAsAtomicUnit=on
  Quantizer : Quantizer  QuantizationInterval=res_gps
  Selector : Selector  InputPortWidth=3  IndexOptions=Index vector (dialog)  Indices=[3]  OutputSizes=1
  Sum : Sum  Inputs=|++
  Switch : Switch  Criteria=u2 > Threshold  Threshold=0.30
  "WGS84toNed " : MATLAB Function  TreatAsAtomicUnit=on
  rumore GPS : RandomNumber  Variance=var_gps  Seed=[18;40;93]  SampleTime=Ts_gps  VectorParams1D=off
  GPS : Outport  VectorParamsAs1DForOutWhenUnconnected=off
  wires:
  Selector/1 -> Switch/2
  rumore GPS/1 -> Sum/2
  Posizione/1 -> "WGS84toNed "/1(posizione)
  "WGS84toNed "/1(posizione_NED) -> Selector/1, Sum/1
  Sum/1 -> Quantizer/1
  MATLAB Function/1(position) -> Switch/3
  Switch/1 -> GPS/1
  Constant/1 -> Switch/1
  Quantizer/1 -> MATLAB Function/1(ned)

== system TeamA_PAsqualo_R19b/Sensors and Environment Models /IMU(giro) ==
  note: rad/s
  omega : Inport  SampleTime=Ts_giroscopio
  Quantizer : Quantizer  QuantizationInterval=res_giroscopio
  Random Number : RandomNumber  Variance=var_giroscopio  Seed=[1; 5; 3]  SampleTime=Ts_giroscopio  VectorParams1D=off
  Sum : Sum  Inputs=|++
  omega_giro : Outport  VectorParamsAs1DForOutWhenUnconnected=off
  wires:
  omega/1 -> Sum/1
  Random Number/1 -> Sum/2
  Sum/1 -> Quantizer/1
  Quantizer/1 -> omega_giro/1

== system TeamA_PAsqualo_R19b/Sensors and Environment Models /Profondimetro ==
  note: metri
  Posizione : Inport  SampleTime=Ts_profondimetro
  Quantizer : Quantizer  QuantizationInterval=res_profondimetro
  Random Number1 : RandomNumber  Variance=var_profondimetro  Seed=85  SampleTime=Ts_profondimetro  VectorParams1D=off
  Selector : Selector  InputPortWidth=3  IndexOptions=Index vector (dialog)  Indices=[ 3]  OutputSizes=1
  Sum1 : Sum  Inputs=|++
  "WGS84toNed " : MATLAB Function  TreatAsAtomicUnit=on
  Profondità : Outport  VectorParamsAs1DForOutWhenUnconnected=off
  wires:
  Posizione/1 -> "WGS84toNed "/1(posizione)
  Selector/1 -> Sum1/1
  Random Number1/1 -> Sum1/2
  "WGS84toNed "/1(posizione_NED) -> Selector/1
  Sum1/1 -> Quantizer/1
  Quantizer/1 -> Profondità/1

== system TeamA_PAsqualo_R19b/Sensors and Environment Models /Sonar_down ==
  Posizione : Inport  SampleTime=Ts_sonar_down
  Orientazione : Inport  Port=2  SampleTime=Ts_sonar_down
  Constant : Constant  Value=tilt_down  VectorParams1D=off  SampleTime=Ts_sonar_down
  Constant1 : Constant  Value=p_sonar_down  VectorParams1D=off  SampleTime=Ts_sonar_down
  MATLAB Function : MATLAB Function  TreatAsAtomicUnit=on
  MATLAB Function1 : MATLAB Function  TreatAsAtomicUnit=on
  Quantizer : Quantizer  QuantizationInterval=res_sonar_down
  Random Number : RandomNumber  Variance=var_sonar_down  SampleTime=Ts_sonar_down  VectorParams1D=off
  Sum : Sum  Inputs=|++
  WGS84toNed 1 : MATLAB Function  TreatAsAtomicUnit=on
  Distanza : Outport  VectorParamsAs1DForOutWhenUnconnected=off
  wires:
  MATLAB Function/2(s_versor_ned) -> MATLAB Function1/2(s_versor_ned)
  WGS84toNed 1/1(posizione_NED) -> MATLAB Function/1(posizione)
  Constant1/1 -> MATLAB Function/4(p_sonar_body)
  MATLAB Function/1(p_sonar_ned) -> MATLAB Function1/1(p_sonar_ned)
  Orientazione/1 -> MATLAB Function/2(orientazione)
  Constant/1 -> MATLAB Function/3(tilt)
  Posizione/1 -> WGS84toNed 1/1(posizione)
  MATLAB Function1/1(sol_t) -> Sum/1
  Random Number/1 -> Sum/2
  Quantizer/1 -> Distanza/1
  Sum/1 -> Quantizer/1

== system TeamA_PAsqualo_R19b/Sensors and Environment Models /Sonar_front ==
  Posizione : Inport  SampleTime=Ts_sonar_front
  Orientazione : Inport  Port=2  SampleTime=Ts_sonar_front
  Constant : Constant  Value=tilt_front  VectorParams1D=off  SampleTime=Ts_sonar_front
  Constant1 : Constant  Value=p_sonar_front  VectorParams1D=off  SampleTime=Ts_sonar_front
  MATLAB Function : MATLAB Function  TreatAsAtomicUnit=on
  MATLAB Function1 : MATLAB Function  TreatAsAtomicUnit=on
  Quantizer : Quantizer  QuantizationInterval=res_sonar_front
  Random Number : RandomNumber  Variance=var_sonar_front  SampleTime=Ts_sonar_front  VectorParams1D=off
  Sum : Sum  Inputs=|++
  WGS84toNed 1 : MATLAB Function  TreatAsAtomicUnit=on
  Distanza : Outport  VectorParamsAs1DForOutWhenUnconnected=off
  wires:
  Posizione/1 -> WGS84toNed 1/1(posizione)
  Constant/1 -> MATLAB Function/3(tilt)
  Orientazione/1 -> MATLAB Function/2(orientazione)
  MATLAB Function/1(p_sonar_ned) -> MATLAB Function1/1(p_sonar_ned)
  Constant1/1 -> MATLAB Function/4(p_sonar_body)
  WGS84toNed 1/1(posizione_NED) -> MATLAB Function/1(posizione)
  MATLAB Function/2(s_versor_ned) -> MATLAB Function1/2(s_versor_ned)
  MATLAB Function1/1(sol_t) -> Sum/1
  Sum/1 -> Quantizer/1
  Random Number/1 -> Sum/2
  Quantizer/1 -> Distanza/1

== system TeamA_PAsqualo_R19b/Sensors and Environment Models /Ultra Short Base Line System ==
  Posizione : Inport  SampleTime=Ts_usbl
  Orientazione : Inport  Port=2  SampleTime=Ts_usbl
  Constant : Constant  Value=p_usbl  VectorParams1D=off
  Constant1 : Constant  Value=p_transponder  VectorParams1D=off
  MATLAB Function1 : MATLAB Function  TreatAsAtomicUnit=on
  MATLAB Function2 : MATLAB Function  TreatAsAtomicUnit=on
  Quantizer : Quantizer  QuantizationInterval=res_usbl
  Random Number : RandomNumber  Variance=var_usbl  Seed=[2; 4; 1]  SampleTime=Ts_usbl  VectorParams1D=off
  Sum : Sum  Inputs=|++
  Vector Concatenate : Concatenate  NumInputs=3  Mode=Multidimensional array
  WGS84toNed 1 : MATLAB Function  TreatAsAtomicUnit=on
  BER : Outport  VectorParamsAs1DForOutWhenUnconnected=off
  wires:
  MATLAB Function2/1(x_t_usbl) -> MATLAB Function1/1(x_t_usbl)
  MATLAB Function1/2(elevation) -> Vector Concatenate/2
  Orientazione/1 -> MATLAB Function2/2(orientazione)
  Constant/1 -> MATLAB Function2/3(p_usbl)
  Constant1/1 -> MATLAB Function2/4(p_transponder)
  Posizione/1 -> WGS84toNed 1/1(posizione)
  MATLAB Function1/3(range) -> Vector Concatenate/3
  MATLAB Function2/2(y_t_usbl) -> MATLAB Function1/2(y_t_usbl)
  WGS84toNed 1/1(posizione_NED) -> MATLAB Function2/1(posizione)
  MATLAB Function2/3(z_t_usbl) -> MATLAB Function1/3(z_t_usbl)
  Vector Concatenate/1 -> Sum/1
  Random Number/1 -> Sum/2
  Quantizer/1 -> BER/1
  Sum/1 -> Quantizer/1
  MATLAB Function1/1(bearing) -> Vector Concatenate/1

== system TeamA_PAsqualo_R19b/Vehicle Model/Thruster A ==
  note: n is the rotational speed of the thruster
      | V is the speed component of the water along the thruster axis
      |
      | n is saturated according to data
      | a dead zone is considered according to data
      | the thruster is characterised by 1st order dynamics (tau = 0.2s)
  n [rad/s] : Inport
  V [m/s] : Inport  Port=2
  Dead Zone : DeadZone  LowerValue=-dead_zone_limit  UpperValue=dead_zone_limit  SaturateOnIntegerOverflow=on
  MATLAB Function : MATLAB Function  TreatAsAtomicUnit=on
  Saturation : Saturate  UpperLimit=n_max  LowerLimit=-n_max
  Transfer Fcn : TransferFcn  Denominator=[0.2 1]
  T i : Outport
  wires:
  V [m/s]/1 -> MATLAB Function/2(V)
  Saturation/1 -> MATLAB Function/1(n)
  Transfer Fcn/1 -> Saturation/1
  Dead Zone/1 -> Transfer Fcn/1
  n [rad/s]/1 -> Dead Zone/1
  MATLAB Function/1(T) -> T i/1

== system TeamA_PAsqualo_R19b/Vehicle Model/Thruster B ==
  note: n is the rotational speed of the thruster
      | V is the speed component of the water along the thruster axis
      |
      | n is saturated according to data
      | a dead zone is considered according to data
      | the thruster is characterised by 1st order dynamics (tau = 0.2s)
  n [rad/s] : Inport
  V [m/s] : Inport  Port=2
  Dead Zone : DeadZone  LowerValue=-dead_zone_limit  UpperValue=dead_zone_limit  SaturateOnIntegerOverflow=on
  MATLAB Function : MATLAB Function  TreatAsAtomicUnit=on
  Saturation : Saturate  UpperLimit=n_max  LowerLimit=-n_max
  Transfer Fcn : TransferFcn  Denominator=[0.2 1]
  T i : Outport
  wires:
  MATLAB Function/1(T) -> T i/1
  n [rad/s]/1 -> Dead Zone/1
  Dead Zone/1 -> Transfer Fcn/1
  Transfer Fcn/1 -> Saturation/1
  Saturation/1 -> MATLAB Function/1(n)
  V [m/s]/1 -> MATLAB Function/2(V)

== system TeamA_PAsqualo_R19b/Vehicle Model/Thruster C ==
  note: n is the rotational speed of the thruster
      | V is the speed component of the water along the thruster axis
      |
      | n is saturated according to data
      | a dead zone is considered according to data
      | the thruster is characterised by 1st order dynamics (tau = 0.2s)
  n [rad/s] : Inport
  V [m/s] : Inport  Port=2
  Dead Zone : DeadZone  LowerValue=-dead_zone_limit  UpperValue=dead_zone_limit  SaturateOnIntegerOverflow=on
  MATLAB Function : MATLAB Function  TreatAsAtomicUnit=on
  Saturation : Saturate  UpperLimit=n_max  LowerLimit=-n_max
  Transfer Fcn : TransferFcn  Denominator=[0.2 1]
  T i : Outport
  wires:
  V [m/s]/1 -> MATLAB Function/2(V)
  Saturation/1 -> MATLAB Function/1(n)
  Transfer Fcn/1 -> Saturation/1
  Dead Zone/1 -> Transfer Fcn/1
  n [rad/s]/1 -> Dead Zone/1
  MATLAB Function/1(T) -> T i/1

== system TeamA_PAsqualo_R19b/Vehicle Model/Thruster D ==
  note: n is the rotational speed of the thruster
      | V is the speed component of the water along the thruster axis
      |
      | n is saturated according to data
      | a dead zone is considered according to data
      | the thruster is characterised by 1st order dynamics (tau = 0.2s)
  n [rad/s] : Inport
  V [m/s] : Inport  Port=2
  Dead Zone : DeadZone  LowerValue=-dead_zone_limit  UpperValue=dead_zone_limit  SaturateOnIntegerOverflow=on
  MATLAB Function : MATLAB Function  TreatAsAtomicUnit=on
  Saturation : Saturate  UpperLimit=n_max  LowerLimit=-n_max
  Transfer Fcn : TransferFcn  Denominator=[0.2 1]
  T i : Outport
  wires:
  MATLAB Function/1(T) -> T i/1
  n [rad/s]/1 -> Dead Zone/1
  Dead Zone/1 -> Transfer Fcn/1
  Transfer Fcn/1 -> Saturation/1
  Saturation/1 -> MATLAB Function/1(n)
  V [m/s]/1 -> MATLAB Function/2(V)

== system TeamA_PAsqualo_R19b/Vehicle Model/Thruster E ==
  note: n is the rotational speed of the thruster
      | V is the speed component of the water along the thruster axis
      |
      | n is saturated according to data
      | a dead zone is considered according to data
      | the thruster is characterised by 1st order dynamics (tau = 0.2s)
  n [rad/s] : Inport
  V [m/s] : Inport  Port=2
  Dead Zone : DeadZone  LowerValue=-dead_zone_limit  UpperValue=dead_zone_limit  SaturateOnIntegerOverflow=on
  MATLAB Function : MATLAB Function  TreatAsAtomicUnit=on
  Saturation : Saturate  UpperLimit=n_max  LowerLimit=-n_max
  Transfer Fcn : TransferFcn  Denominator=[0.2 1]
  T i : Outport
  wires:
  V [m/s]/1 -> MATLAB Function/2(V)
  Saturation/1 -> MATLAB Function/1(n)
  Transfer Fcn/1 -> Saturation/1
  Dead Zone/1 -> Transfer Fcn/1
  n [rad/s]/1 -> Dead Zone/1
  MATLAB Function/1(T) -> T i/1

== system TeamA_PAsqualo_R19b/Vehicle Model/Thruster F ==
  note: n is the rotational speed of the thruster
      | V is the speed component of the water along the thruster axis
      |
      | n is saturated according to data
      | a dead zone is considered according to data
      | the thruster is characterised by 1st order dynamics (tau = 0.2s)
  n [rad/s] : Inport
  V [m/s] : Inport  Port=2
  Dead Zone : DeadZone  LowerValue=-dead_zone_limit  UpperValue=dead_zone_limit  SaturateOnIntegerOverflow=on
  MATLAB Function : MATLAB Function  TreatAsAtomicUnit=on
  Saturation : Saturate  UpperLimit=n_max  LowerLimit=-n_max
  Transfer Fcn : TransferFcn  Denominator=[0.2 1]
  T i : Outport
  wires:
  MATLAB Function/1(T) -> T i/1
  n [rad/s]/1 -> Dead Zone/1
  Dead Zone/1 -> Transfer Fcn/1
  Transfer Fcn/1 -> Saturation/1
  Saturation/1 -> MATLAB Function/1(n)
  V [m/s]/1 -> MATLAB Function/2(V)

== system TeamA_PAsqualo_R19b/Vehicle Model/Thruster G ==
  note: n is the rotational speed of the thruster
      | V is the speed component of the water along the thruster axis
      |
      | n is saturated according to data
      | a dead zone is considered according to data
      | the thruster is characterised by 1st order dynamics (tau = 0.2s)
  n [rad/s] : Inport
  V [m/s] : Inport  Port=2
  Dead Zone : DeadZone  LowerValue=-dead_zone_limit  UpperValue=dead_zone_limit  SaturateOnIntegerOverflow=on
  MATLAB Function : MATLAB Function  TreatAsAtomicUnit=on
  Saturation : Saturate  UpperLimit=n_max  LowerLimit=-n_max
  Transfer Fcn : TransferFcn  Denominator=[0.2 1]
  T i : Outport
  wires:
  V [m/s]/1 -> MATLAB Function/2(V)
  Saturation/1 -> MATLAB Function/1(n)
  Transfer Fcn/1 -> Saturation/1
  Dead Zone/1 -> Transfer Fcn/1
  n [rad/s]/1 -> Dead Zone/1
  MATLAB Function/1(T) -> T i/1

== system TeamA_PAsqualo_R19b/controller1/abort mission ==
  enable : Inport
  references : Inport  Port=2
  est_state : Inport  Port=3
  abort mission : MATLAB Function  TreatAsAtomicUnit=on
  abort : Outport
  wires:
  enable/1 -> abort mission/1(enable)
  references/1 -> abort mission/2(ref)
  est_state/1 -> abort mission/3(est_meas)
  abort mission/1(abort) -> abort/1

== system TeamA_PAsqualo_R19b/controller1/diving controller ==
  enable : Inport
  references : Inport  Port=2
  est_state : Inport  Port=3
  Mux : Mux  Inputs=6
  heave_controller : Subsystem
  pitch_controller : Subsystem
  roll_controller : Subsystem
  surge_controller : Subsystem
  sway_controller : Subsystem
  yaw_controller : Subsystem
  tau_div : Outport
  wires:
  sway_controller/1(Y) -> Mux/2  "Y"
  yaw_controller/1(N) -> Mux/6  "N"
  Mux/1 -> tau_div/1
  heave_controller/1(Z) -> Mux/3  "Z"
  references/1 -> surge_controller/2(references), heave_controller/2(references), roll_controller/2(references), yaw_controller/2(references), pitch_controller/2(references), sway_controller/2(references)
  est_state/1 -> sway_controller/3("estimated measures "), heave_controller/3("estimated measures "), roll_controller/3("estimated measures "), yaw_controller/3("estimated measures "), pitch_controller/3("estimated measures "), surge_controller/3("estimated measures ")
  surge_controller/1(X) -> Mux/1  "X"
  roll_controller/1(K) -> Mux/4  "K"
  pitch_controller/1(M) -> Mux/5  "M"
  enable/1 -> sway_controller/1(enable), heave_controller/1(enable), yaw_controller/1(enable), pitch_controller/1(enable), roll_controller/1(enable), surge_controller/1(enable)

== system TeamA_PAsqualo_R19b/controller1/positioning controller ==
  enable : Inport
  references : Inport  Port=2
  est_state : Inport  Port=3
  Mux : Mux  Inputs=6
  heave_controller : Subsystem
  pitch_controller : Subsystem
  roll_controller : Subsystem
  surge_controller : Subsystem
  sway_controller : Subsystem
  yaw_controller : Subsystem
  tau_pos : Outport
  wires:
  enable/1 -> sway_controller/1(enable), heave_controller/1(enable), yaw_controller/1(enable), pitch_controller/1(enable), roll_controller/1(enable), surge_controller/1(enable)
  yaw_controller/1(N) -> Mux/6  "N"
  references/1 -> surge_controller/2(references), heave_controller/2(references), roll_controller/2(references), yaw_controller/2(references), pitch_controller/2(references), sway_controller/2(references)
  pitch_controller/1(M) -> Mux/5  "M"
  est_state/1 -> sway_controller/3("estimated measures "), heave_controller/3("estimated measures "), roll_controller/3("estimated measures "), yaw_controller/3("estimated measures "), pitch_controller/3("estimated measures "), surge_controller/3("estimated measures ")
  surge_controller/1(X) -> Mux/1  "X"
  sway_controller/1(Y) -> Mux/2  "Y"
  roll_controller/1(K) -> Mux/4  "K"
  Mux/1 -> tau_pos/1
  heave_controller/1(Z) -> Mux/3  "Z"
